simulink model "Figure_MPCNonModual"  (R2015b)
settings: Solver=ode4  StartTime=0.0  StopTime=TMax  FixedStep=Ts  RelTol=1e-3
values from neighbouring files (symbols this model uses):
  DT = fscanf(fid,'    [YY_Read_FAST_Input.m]
  NDOF = 24    [YY_Read_FAST_Input.m]
  NumOuts = 2    [Reduced4to3_2DOF_18.mat]    (also in YY_Read_FAST_Input.m = 1)
  OutList = {}    [YY_Read_FAST_Input.m]
  q_init = zeros(1,NDOF)    [YY_Read_FAST_Input.m]
  qdot_init = zeros(1,NDOF)    [YY_Read_FAST_Input.m]
undefined symbols (not defined in the file or in its folder): strmatch
libraries: mpclib x1
settings Model: Creator=yuy13010  LastModifiedBy=yuy13010

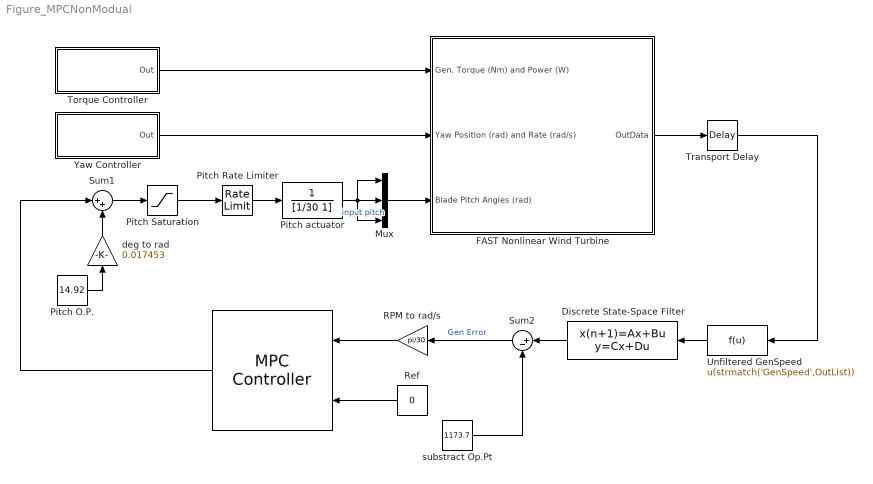
== system Figure_MPCNonModual ==
  " " : mpclib/MPC Controller  SCDEnableBlockLinearizationSpecification=on  mpcobj=mpcobj  x0=[]  is_multiple=0  enable_value=0  return_u0=off  ref_from_ws=off  ref_signal_name=[]  ref_preview=off  md_from_ws=off  md_signal_name=[]  md_preview=off  from_project=off  project_file=MPCtask.mat  md_inport=off  mv_inport=off  cost_outport=off  return_sequence=off  return_qpstatus=off  return_state=off  state_inport=off  lims_inport=off  ywt_inport=off  is_designfromscratch=0  uwt_inport=off  duwt_inport=off  rhoeps_inport=off  uref_inport=off  n_ts=0.0125  n_mv=1  n_md=0  n_ud=0  n_mo=1  n_uo=0  BlockDataType=double  SampleTimeInherited=off  switch_inport=off
  Discrete State-Space Filter : DiscreteStateSpace  A=0.9806  B=0.0194  C=0.9806  D=0.0194  SampleTime=DT
  FAST Nonlinear Wind Turbine : Subsystem
  Mux : Mux  Inputs=3
  Pitch O.P. : Constant  Value=14.92
  Pitch Rate Limiter : RateLimiter  RisingSlewLimit=0.1396263  FallingSlewLimit=-0.1396263  SampleTimeMode=inherited
  Pitch Saturation : Saturate  UpperLimit=1.570796  LowerLimit=0  SampleTime=DT
  Pitch actuator : TransferFcn  Denominator=[1/30 1]
  RPM to rad/s : Gain  Gain=pi/30  SaturateOnIntegerOverflow=on  OutDataTypeStr=Inherit: Same as input  ParamDataTypeStr=Inherit: Same as input
  Ref : Constant  Value=0
  Sum1 : Sum  Inputs=|++
  Sum2 : Sum  Inputs=|+-  SampleTime=DT
  Torque Controller : Subsystem
  Transport Delay : TransportDelay  DelayTime=0.02
  Unfiltered GenSpeed : Fcn  Expr=u(strmatch('GenSpeed',OutList))  SampleTime=DT
  Yaw Controller : Subsystem
  deg to rad : Gain  Gain=0.017453  SaturateOnIntegerOverflow=on  OutDataTypeStr=Inherit: Same as input  ParamDataTypeStr=Inherit: Same as input
  substract Op.Pt : Constant  Value=1173.7
  wires:
  Torque Controller/1(Out) -> FAST Nonlinear Wind Turbine/1(Gen. Torque (Nm) and Power (W))
  Yaw Controller/1(Out) -> FAST Nonlinear Wind Turbine/2(Yaw Position (rad) and Rate (rad/s))
  Mux/1 -> FAST Nonlinear Wind Turbine/3(Blade Pitch Angles (rad))
  substract Op.Pt/1 -> Sum2/2
  Unfiltered GenSpeed/1 -> Discrete State-Space Filter/1
  Discrete State-Space Filter/1 -> Sum2/1
  FAST Nonlinear Wind Turbine/1(OutData) -> Transport Delay/1
  Transport Delay/1 -> Unfiltered GenSpeed/1
  Pitch O.P./1 -> deg to rad/1
  deg to rad/1 -> Sum1/2
  Sum1/1 -> Pitch Saturation/1
  Pitch Saturation/1 -> Pitch Rate Limiter/1
  Pitch Rate Limiter/1 -> Pitch actuator/1
  " "/1 -> Sum1/1
  Ref/1 -> " "/2
  RPM to rad/s/1 -> " "/1
  Pitch actuator/1 -> Mux/1, Mux/3, Mux/2  "input pitch"
  Sum2/1 -> RPM to rad/s/1  "Gen Error"

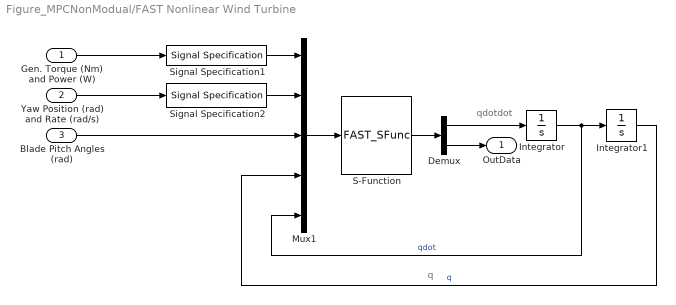
== system Figure_MPCNonModual/FAST Nonlinear Wind Turbine ==
  note: qdotdot
  note: q
  Gen. Torque (Nm) and Power (W) : Inport
  Yaw Position (rad) and Rate (rad/s) : Inport  Port=2
  Blade Pitch Angles (rad) : Inport  Port=3
  Demux : Demux  Outputs=[NDOF, NumOuts]
  Integrator : Integrator  InitialCondition=qdot_init
  Integrator1 : Integrator  InitialCondition=q_init
  Mux1 : Mux  Inputs=5
  S-Function : S-Function  FunctionName=FAST_SFunc  SFunctionDeploymentMode=off  EnableBusSupport=off
  Signal Specification1 : SignalSpecification  OutDataTypeStr=double  Dimensions=2
  Signal Specification2 : SignalSpecification  OutDataTypeStr=double  Dimensions=2
  OutData : Outport
  wires:
  Integrator/1 -> Integrator1/1, Mux1/5  "qdot"
  Gen. Torque (Nm) and Power (W)/1 -> Signal Specification1/1
  S-Function/1 -> Demux/1
  Demux/1 -> Integrator/1
  Demux/2 -> OutData/1
  Mux1/1 -> S-Function/1
  Blade Pitch Angles (rad)/1 -> Mux1/3
  Yaw Position (rad) and Rate (rad/s)/1 -> Signal Specification2/1
  Integrator1/1 -> Mux1/4  "q"
  Signal Specification1/1 -> Mux1/1
  Signal Specification2/1 -> Mux1/2

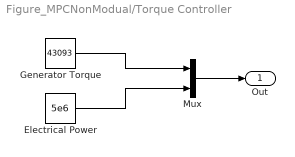
== system Figure_MPCNonModual/Torque Controller ==
  Electrical Power : Constant  Value=5e6
  Generator Torque : Constant  Value=43093
  Mux : Mux  Inputs=2
  Out : Outport
  wires:
  Mux/1 -> Out/1
  Generator Torque/1 -> Mux/1
  Electrical Power/1 -> Mux/2

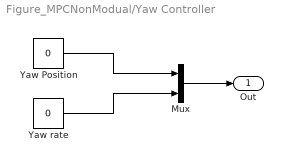
== system Figure_MPCNonModual/Yaw Controller ==
  Mux : Mux  Inputs=2
  Yaw Position : Constant  Value=0
  Yaw rate : Constant  Value=0
  Out : Outport
  wires:
  Mux/1 -> Out/1
  Yaw Position/1 -> Mux/1
  Yaw rate/1 -> Mux/2
